simulink model "sampleModel1700"  (R2023a)
settings: Solver=VariableStepAuto  StartTime=0.0  StopTime=10.0  RelTol=1e-3
libraries: hdlsllib x8, simulink x3
settings Model: Creator=user1  LastModifiedBy=user1

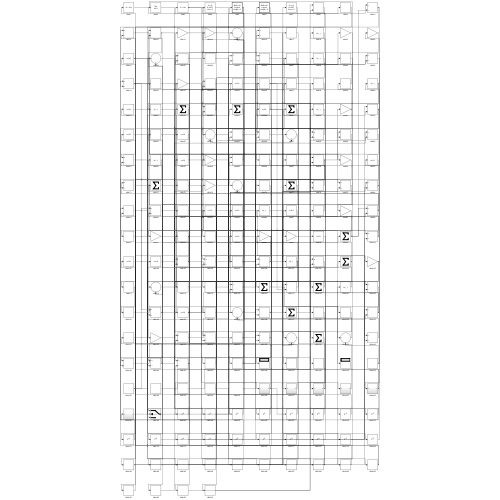
[thumbnail: Simulink's stored preview of the top-level diagram]
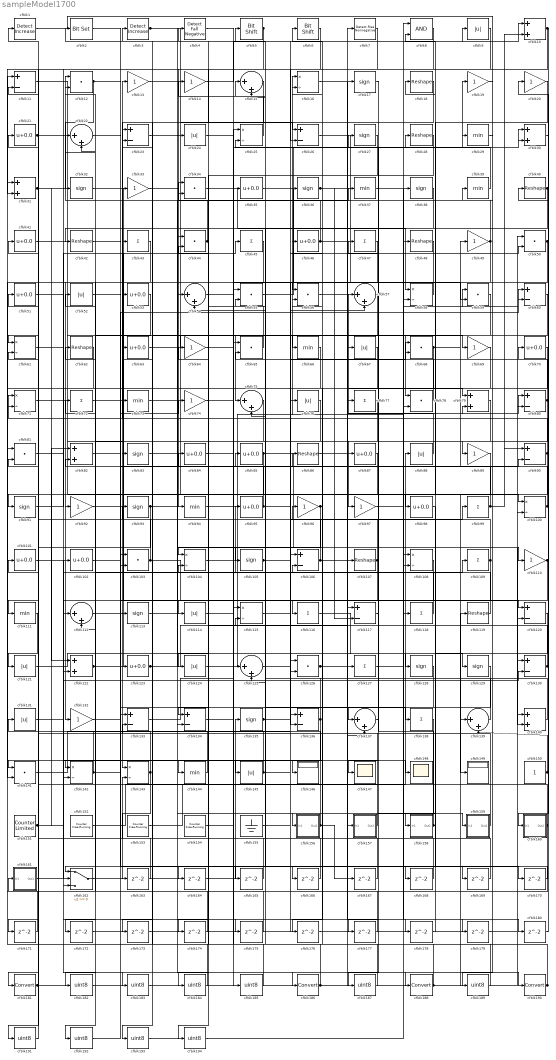
== system sampleModel1700 ==
  cfblk1 : simulink/Logic and Bit Operations/Detect Increase  vinit=0.0  OutDataTypeStr=boolean
      settings: LibrarySourceBlock=|
      | hdlsllib/Logic and Bit
      | Operations/Detect
      | Increase
  cfblk{10,30..31,79,82,122,140} (7 alike) : Sum
  cfblk{16,25,58,61,71,100,104,108,115,142..143} (11 alike) : Product  Inputs=*/  RndMeth=Zero  SaturateOnIntegerOverflow=on
  cfblk{21,35,41,46,51,53,63,70,84..85,87,95,98,101..102,123} (16 alike) : Bias  Bias=0.0  SaturateOnIntegerOverflow=off
  cfblk{12,34,44,50,55..56,59,65,68,78,81,103,126,141} (14 alike) : DotProduct  OutDataTypeStr=Inherit: Inherit via internal rule
  cfblk{17,27,32,36,38,83,91,93,105,113,128..129,135} (13 alike) : Signum
  cfblk{11,23,26,60,80,90,106,117,120,130,133..134,136} (13 alike) : Sum  Inputs=+-
  cfblk{18,28,40,42,48,62,86,107,119} (9 alike) : Reshape
  cfblk{43,45,47,72,77,99,109,116,118,127,138} (11 alike) : Sum  Inputs=+
  cfblk{13..14,19..20,33,49,64,69,74,89,92,96..97,110,132} (15 alike) : Gain
  cfblk{29,37,39,66,73,94,111,144} (8 alike) : MinMax
  cfblk{15,22,54,57,75,112,125,137,139} (9 alike) : Sum  Inputs=|++
  cfblk{9,24,52,67,76,88,114,121,124,131,145} (11 alike) : Abs  SaturateOnIntegerOverflow=off
  cfblk146 : Display
  cfblk147 : Scope
  cfblk148 : Scope
  cfblk149 : Display
  cfblk150 : Constant  SampleTime=-1
  cfblk151 : hdlsllib/Sources/Counter Limited  uplimit=7  tsamp=-1
  cfblk152 : hdlsllib/Sources/Counter Free-Running  NumBits=16  tsamp=-1
  cfblk153 : hdlsllib/Sources/Counter Free-Running  NumBits=16  tsamp=-1
  cfblk154 : hdlsllib/Sources/Counter Free-Running  NumBits=16  tsamp=-1
  cfblk155 : Ground
  cfblk156 : Subsystem
      settings: LibrarySourceBlock=|
      | hdlsllib/Ports &
      | Subsystems/Subsystem
  cfblk157 : Subsystem
      settings: LibrarySourceBlock=|
      | hdlsllib/Ports &
      | Subsystems/Subsystem
  cfblk158 : Subsystem
      settings: LibrarySourceBlock=|
      | hdlsllib/Ports &
      | Subsystems/Subsystem
  cfblk159 : Subsystem
      settings: LibrarySourceBlock=|
      | hdlsllib/Ports &
      | Subsystems/Subsystem
  cfblk160 : Subsystem
      settings: LibrarySourceBlock=|
      | hdlsllib/Ports &
      | Subsystems/Subsystem
  cfblk161 : Subsystem
      settings: LibrarySourceBlock=|
      | hdlsllib/Ports &
      | Subsystems/Subsystem
  cfblk162 : Switch  SaturateOnIntegerOverflow=off  InputSameDT=off
  cfblk{163..180} (18 alike) : Delay  SampleTime=1
  cfblk{181,186,188,190} (4 alike) : DataTypeConversion  SaturateOnIntegerOverflow=off  RndMeth=Floor
  cfblk{182..185,187,189,191..194} (10 alike) : DataTypeConversion  OutDataTypeStr=uint8  SaturateOnIntegerOverflow=off  RndMeth=Floor
  cfblk2 : simulink/Logic and Bit Operations/Bit Set  iBit=0
      settings: LibrarySourceBlock=|
      | hdlsllib/Logic and Bit
      | Operations/Bit Set
  cfblk3 : simulink/Logic and Bit Operations/Detect Increase  vinit=0.0  OutDataTypeStr=boolean
      settings: LibrarySourceBlock=|
      | hdlsllib/Logic and Bit
      | Operations/Detect
      | Increase
  cfblk4 : hdlsllib/Logic and Bit Operations/Detect Fall Negative  vinit=0  OutDataTypeStr=boolean
  cfblk5 : hdlsllib/Logic and Bit Operations/Bit Shift  mode=Shift Left Logical  N=0
  cfblk6 : hdlsllib/Logic and Bit Operations/Bit Shift  mode=Shift Left Logical  N=0
  cfblk7 : hdlsllib/Logic and Bit Operations/Detect Rise Nonnegative  vinit=0  OutDataTypeStr=boolean
  cfblk8 : Logic  AllPortsSameDT=off  OutDataTypeStr=boolean
  wires:
  cfblk88/1 -> cfblk57/1
  cfblk153/1 -> cfblk88/1
  cfblk90/1 -> cfblk132/1, cfblk73/1, cfblk71/1
  cfblk121/1 -> cfblk128/1
  cfblk93/1 -> cfblk36/1, cfblk191/1
  cfblk110/1 -> cfblk140/2, cfblk184/1
  cfblk46/1 -> cfblk107/1, cfblk78/2, cfblk12/2
  cfblk15/1 -> cfblk143/1
  cfblk39/1 -> cfblk5/1
  cfblk106/1 -> cfblk80/1, cfblk23/2
  cfblk98/1 -> cfblk158/1(In1)
  cfblk122/1 -> cfblk45/1, cfblk22/2
  cfblk127/1 -> cfblk59/1
  cfblk142/1 -> cfblk21/1, cfblk86/1
  cfblk5/1 -> cfblk94/1, cfblk61/1
  cfblk1/1 -> cfblk39/1
  cfblk65/1 -> cfblk2/1
  cfblk47/1 -> cfblk92/1
  cfblk77/1 -> cfblk97/1
  cfblk17/1 -> cfblk137/1
  cfblk7/1 -> cfblk181/1
  cfblk62/1 -> cfblk111/1
  cfblk60/1 -> cfblk75/1
  cfblk20/1 -> cfblk98/1
  cfblk51/1 -> cfblk112/1
  cfblk10/1 -> cfblk70/1, cfblk162/3
  cfblk129/1 -> cfblk147/1
  cfblk72/1 -> cfblk13/1
  cfblk26/1 -> cfblk118/1
  cfblk29/1 -> cfblk89/1
  cfblk34/1 -> cfblk58/1
  cfblk152/1 -> cfblk38/1
  cfblk124/1 -> cfblk16/1
  cfblk117/1 -> cfblk47/1
  cfblk32/1 -> cfblk114/1
  cfblk123/1 -> cfblk67/1, cfblk90/2
  cfblk3/1 -> cfblk26/1, cfblk110/1
  cfblk94/1 -> cfblk8/1
  cfblk13/1 -> cfblk157/1(In1)
  cfblk140/1 -> cfblk4/1
  cfblk130/1 -> cfblk27/1, cfblk34/2
  cfblk113/1 -> cfblk156/1(In1)
  cfblk21/1 -> cfblk83/1, cfblk178/1
  cfblk107/1 -> cfblk62/1, cfblk134/2, cfblk122/2, cfblk104/2
  cfblk162/1 -> cfblk135/1
  cfblk58/1 -> cfblk54/1
  cfblk41/1 -> cfblk78/1
  cfblk63/1 -> cfblk69/1
  cfblk56/1 -> cfblk17/1
  cfblk109/1 -> cfblk34/1, cfblk142/2
  cfblk114/1 -> cfblk35/1
  cfblk22/1 -> cfblk123/1
  cfblk118/1 -> cfblk16/2
  cfblk27/1 -> cfblk44/1
  cfblk96/1 -> cfblk146/1, cfblk104/1
  cfblk82/1 -> cfblk74/1
  cfblk101/1 -> cfblk190/1
  cfblk61/1 -> cfblk162/2
  cfblk136/1 -> cfblk141/1, cfblk54/2
  cfblk44/1 -> cfblk12/1, cfblk42/1
  cfblk16/1 -> cfblk129/1
  cfblk85/1 -> cfblk140/1, cfblk91/1
  cfblk71/1 -> cfblk127/1
  cfblk53/1 -> cfblk112/2
  cfblk141/1 -> cfblk76/1
  cfblk105/1 -> cfblk57/2, cfblk99/1
  cfblk145/1 -> cfblk68/1, cfblk30/2, cfblk3/1
  cfblk80/1 -> cfblk15/1, cfblk145/1
  cfblk11/1 -> cfblk66/1
  cfblk25/1 -> cfblk14/1
  cfblk91/1 -> cfblk43/1
  cfblk111/1 -> cfblk121/1
  cfblk103/1 -> cfblk51/1, cfblk137/2
  cfblk14/1 -> cfblk9/1
  cfblk70/1 -> cfblk116/1
  cfblk30/1 -> cfblk160/1(In1)
  cfblk160/1(Out1) -> cfblk161/1(In1), cfblk25/2, cfblk11/2
  cfblk119/1 -> cfblk72/1
  cfblk139/1 -> cfblk96/1
  cfblk31/1 -> cfblk115/1, cfblk122/1, cfblk148/1
  cfblk9/1 -> cfblk26/2
  cfblk126/1 -> cfblk106/2, cfblk79/2
  cfblk131/1 -> cfblk109/1
  cfblk37/1 -> cfblk100/1
  cfblk161/1(Out1) -> cfblk130/2
  cfblk150/1 -> cfblk40/1, cfblk139/2
  cfblk92/1 -> cfblk49/1
  cfblk24/1 -> cfblk125/1
  cfblk8/1 -> cfblk31/2
  cfblk104/1 -> cfblk48/1
  cfblk12/1 -> cfblk32/1, cfblk120/2
  cfblk112/1 -> cfblk95/1
  cfblk115/1 -> cfblk50/2
  cfblk55/1 -> cfblk19/1
  cfblk116/1 -> cfblk149/1
  cfblk50/1 -> cfblk126/2, cfblk194/1
  cfblk6/1 -> cfblk24/1
  cfblk68/1 -> cfblk60/1, cfblk105/1, cfblk71/2
  cfblk74/1 -> cfblk25/1
  cfblk40/1 -> cfblk125/2, cfblk193/1
  cfblk99/1 -> cfblk18/1, cfblk10/2, cfblk90/1
  cfblk18/1 -> cfblk53/1
  cfblk43/1 -> cfblk103/2
  cfblk143/1 -> cfblk61/2, cfblk163/1
  cfblk159/1(Out1) -> cfblk41/1
  cfblk73/1 -> cfblk120/1
  cfblk95/1 -> cfblk10/1, cfblk82/2
  cfblk83/1 -> cfblk139/1
  cfblk57/1 -> cfblk124/1
  cfblk102/1 -> cfblk85/1
  cfblk132/1 -> cfblk60/2
  cfblk155/1 -> cfblk136/1
  cfblk157/1(Out1) -> cfblk133/2
  cfblk36/1 -> cfblk58/2, cfblk117/2, cfblk79/1
  cfblk35/1 -> cfblk59/2
  cfblk52/1 -> cfblk138/1
  cfblk38/1 -> cfblk75/2
  cfblk89/1 -> cfblk136/2
  cfblk144/1 -> cfblk93/1
  cfblk64/1 -> cfblk188/1
  cfblk28/1 -> cfblk144/1
  cfblk135/1 -> cfblk55/2, cfblk28/1
  cfblk78/1 -> cfblk6/1
  cfblk125/1 -> cfblk29/1
  cfblk133/1 -> cfblk37/1
  cfblk76/1 -> cfblk134/1
  cfblk59/1 -> cfblk113/1
  cfblk158/1(Out1) -> cfblk68/2, cfblk77/1
  cfblk134/1 -> cfblk30/1
  cfblk33/1 -> cfblk186/1
  cfblk100/1 -> cfblk46/1, cfblk52/1
  cfblk48/1 -> cfblk141/2
  cfblk156/1(Out1) -> cfblk63/1, cfblk167/1
  cfblk79/1 -> cfblk142/1
  cfblk4/1 -> cfblk56/1
  cfblk84/1 -> cfblk159/1(In1)
  cfblk49/1 -> cfblk23/1, cfblk174/1
  cfblk151/1 -> cfblk102/1, cfblk82/1
  cfblk163/1 -> cfblk1/1
  cfblk2/1 -> cfblk164/1
  cfblk164/1 -> cfblk55/1
  cfblk128/1 -> cfblk165/1
  cfblk165/1 -> cfblk133/1
  cfblk69/1 -> cfblk166/1
  cfblk166/1 -> cfblk143/2
  cfblk167/1 -> cfblk115/2
  cfblk120/1 -> cfblk168/1
  cfblk168/1 -> cfblk15/2
  cfblk42/1 -> cfblk169/1
  cfblk169/1 -> cfblk44/2
  cfblk54/1 -> cfblk170/1
  cfblk170/1 -> cfblk162/1
  cfblk66/1 -> cfblk171/1
  cfblk171/1 -> cfblk11/1
  cfblk45/1 -> cfblk172/1
  cfblk172/1 -> cfblk80/2
  cfblk67/1 -> cfblk173/1
  cfblk173/1 -> cfblk126/1
  cfblk174/1 -> cfblk22/1
  cfblk23/1 -> cfblk175/1
  cfblk175/1 -> cfblk31/1
  cfblk87/1 -> cfblk176/1
  cfblk176/1 -> cfblk100/2
  cfblk138/1 -> cfblk177/1
  cfblk177/1 -> cfblk106/1
  cfblk178/1 -> cfblk8/2
  cfblk86/1 -> cfblk179/1
  cfblk179/1 -> cfblk50/1
  cfblk97/1 -> cfblk180/1
  cfblk180/1 -> cfblk20/1
  cfblk181/1 -> cfblk87/1, cfblk117/1
  cfblk75/1 -> cfblk182/1
  cfblk182/1 -> cfblk7/1
  cfblk81/1 -> cfblk183/1
  cfblk183/1 -> cfblk130/1
  cfblk184/1 -> cfblk81/1
  cfblk154/1 -> cfblk185/1
  cfblk185/1 -> cfblk81/2
  cfblk186/1 -> cfblk65/2, cfblk119/1
  cfblk137/1 -> cfblk187/1
  cfblk187/1 -> cfblk33/1
  cfblk188/1 -> cfblk56/2, cfblk65/1
  cfblk19/1 -> cfblk189/1
  cfblk189/1 -> cfblk64/1
  cfblk190/1 -> cfblk84/1, cfblk131/1
  cfblk191/1 -> cfblk101/1
  cfblk108/1 -> cfblk192/1
  cfblk192/1 -> cfblk103/1
  cfblk193/1 -> cfblk108/1
  cfblk194/1 -> cfblk108/2

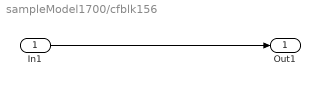
== system sampleModel1700/cfblk156 ==
  In1 : Inport
  Out1 : Outport
  wires:
  In1/1 -> Out1/1

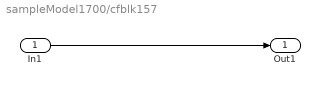
== system sampleModel1700/cfblk157 ==
  In1 : Inport
  Out1 : Outport
  wires:
  In1/1 -> Out1/1

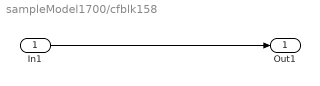
== system sampleModel1700/cfblk158 ==
  In1 : Inport
  Out1 : Outport
  wires:
  In1/1 -> Out1/1

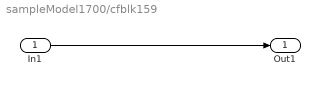
== system sampleModel1700/cfblk159 ==
  In1 : Inport
  Out1 : Outport
  wires:
  In1/1 -> Out1/1

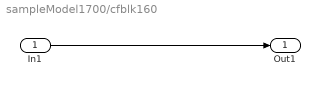
== system sampleModel1700/cfblk160 ==
  In1 : Inport
  Out1 : Outport
  wires:
  In1/1 -> Out1/1

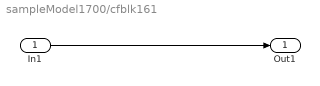
== system sampleModel1700/cfblk161 ==
  In1 : Inport
  Out1 : Outport
  wires:
  In1/1 -> Out1/1
